simulink model "lets_go"  (R2020b)
settings: Solver=VariableStepAuto  StartTime=0.0  StopTime=10.0  RelTol=1e-3
values from neighbouring files (symbols this model uses):
  A_2 = zeros(3)    [Trial_Script.m]
  B_2 = I_inv    [Trial_Script.m]
  C_2 = eye(3)    [Trial_Script.m]
  D_2 = zeros(3)    [Trial_Script.m]
libraries: mpclib x1, cstblocks x1
settings Model: Creator=Jonathan van Zyl  LastModifiedBy=Jonathan van Zyl

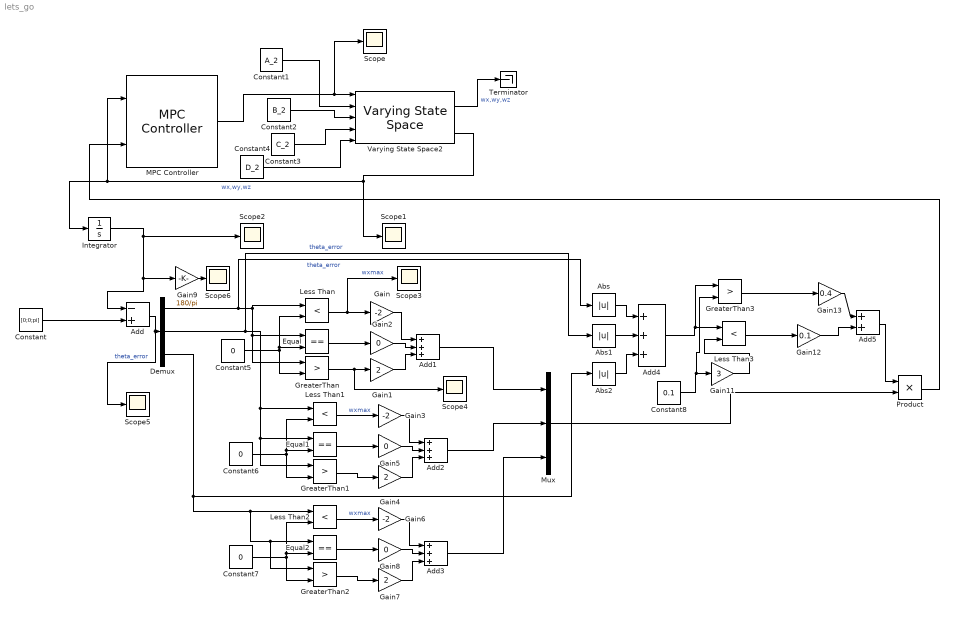
== system lets_go ==
  Abs : Abs
  Abs1 : Abs
  Abs2 : Abs
  Add : Sum  Inputs=-+
  Add{1..4} (4 alike) : Sum  Inputs=+++
  Add5 : Sum
  Constant : Constant  Value=[0;0;pi]
  Constant1 : Constant  Value=A_2
  Constant2 : Constant  Value=B_2
  Constant3 : Constant  Value=C_2
  Constant4 : Constant  Value=D_2
  Constant5 : Constant  Value=0
  Constant6 : Constant  Value=0
  Constant7 : Constant  Value=0
  Constant8 : Constant  Value=0.1
  Demux : Demux  Outputs=3
  Equal : RelationalOperator  Operator===  OutDataTypeStr=boolean  RndMeth=Simplest
  Equal1 : RelationalOperator  Operator===  OutDataTypeStr=boolean  RndMeth=Simplest
  Equal2 : RelationalOperator  Operator===  OutDataTypeStr=boolean  RndMeth=Simplest
  Gain : Gain  Gain=-2
  Gain1 : Gain  Gain=2
  Gain11 : Gain  Gain=3
  Gain12 : Gain  Gain=0.1
  Gain13 : Gain  Gain=0.4
  Gain2 : Gain  Gain=0
  Gain3 : Gain  Gain=-2
  Gain4 : Gain  Gain=2
  Gain5 : Gain  Gain=0
  Gain6 : Gain  Gain=-2
  Gain7 : Gain  Gain=2
  Gain8 : Gain  Gain=0
  Gain9 : Gain  Gain=180/pi
  GreaterThan{,1..3} (4 alike) : RelationalOperator  Operator=>  OutDataTypeStr=boolean  RndMeth=Simplest
  Integrator : Integrator
  Less Than{,1..3} (4 alike) : RelationalOperator  Operator=<  OutDataTypeStr=boolean  RndMeth=Simplest
  MPC Controller : mpclib/MPC Controller  SCDEnableBlockLinearizationSpecification=on  mpcobj=mpc1  is_multiple=0  enable_value=0  return_u0=off  updateMPCinCallerWorkspace=on  md_inport=off  mv_inport=off  uref_inport=off  return_cost=off  return_mvseq=off  return_qpstatus=off  return_xseq=off  return_state=off  return_ovseq=off  state_inport=off  umin_inport=off  umax_inport=off  ymin_inport=off  ymax_inport=off  cc_inport=off  ywt_inport=off  uwt_inport=off  duwt_inport=off  rhoeps_inport=off  pm_inport=off  MaximumP=10  HorizonChoice=FixedHorizon  n_ts=0.1  n_p=10  n_mv=3  n_md=0  n_ud=0  n_mo=3  n_uo=0  BlockDataType=double  SampleTimeInherited=off  switch_inport=off
  Mux : Mux  Inputs=3
  Product : Product
  Scope{,1..6} (7 alike) : Scope
  Terminator : Terminator
  Varying State Space2 : cstblocks/Linear Parameter Varying/Varying State Space  x0=0  xNames=''  OutputX=on  OutputDX=off
  wires:
  Product/1 -> MPC Controller/2
  Gain9/1 -> Scope6/1
  Mux/1 -> Product/2
  Add3/1 -> Mux/3
  Gain1/1 -> Add1/3
  Gain6/1 -> Add3/1
  Gain5/1 -> Add2/2
  Add2/1 -> Mux/2
  Integrator/1 -> Gain9/1, Add/1, Scope2/1
  Constant1/1 -> Varying State Space2/2
  GreaterThan1/1 -> Gain4/1
  Equal/1 -> Gain2/1
  GreaterThan/1 -> Scope4/1, Gain1/1
  Equal2/1 -> Gain8/1
  Equal1/1 -> Gain5/1
  Demux/2 -> Abs1/1, GreaterThan1/1, Equal1/1, Less Than1/1  "theta_error"
  Gain2/1 -> Add1/2
  Gain7/1 -> Add3/3
  Gain/1 -> Add1/1
  Gain4/1 -> Add2/3
  Constant6/1 -> Equal1/2, Less Than1/2, GreaterThan1/2
  Less Than1/1 -> Gain3/1  "wxmax"
  Constant7/1 -> Equal2/2, Less Than2/2, GreaterThan2/2
  Gain8/1 -> Add3/2
  Gain3/1 -> Add2/1
  Demux/1 -> Abs/1, GreaterThan/1, Equal/1, Less Than/1  "theta_error"
  Add1/1 -> Mux/1
  Constant5/1 -> Equal/2, Less Than/2, GreaterThan/2
  GreaterThan2/1 -> Gain7/1
  Less Than/1 -> Scope3/1, Gain/1  "wxmax"
  Add/1 -> Scope5/1, Demux/1  "theta_error"
  Varying State Space2/1 -> Terminator/1  "wx,wy,wz"
  Constant2/1 -> Varying State Space2/3
  Less Than2/1 -> Gain6/1  "wxmax"
  Constant4/1 -> Varying State Space2/5
  Varying State Space2/2 -> Scope1/1, Integrator/1, MPC Controller/1  "wx,wy,wz"
  MPC Controller/1 -> Varying State Space2/1, Scope/1
  Constant/1 -> Add/2
  Constant3/1 -> Varying State Space2/4
  Demux/3 -> Abs2/1, GreaterThan2/1, Equal2/1, Less Than2/1
  Abs/1 -> Add4/1
  Abs1/1 -> Add4/2
  Abs2/1 -> Add4/3
  Add4/1 -> GreaterThan3/1, Less Than3/1
  Constant8/1 -> GreaterThan3/2, Gain11/1
  Gain11/1 -> Less Than3/2
  Less Than3/1 -> Gain12/1
  GreaterThan3/1 -> Gain13/1
  Gain13/1 -> Add5/1
  Gain12/1 -> Add5/2
  Add5/1 -> Product/1
